simulink model "control_experiment"  (R2023b)
settings: Solver=VariableStepAuto  StartTime=0.0  StopTime=40  MaxStep=1e-4  RelTol=1e-3
values from neighbouring files (symbols this model uses):
  Bp_ = 1.25e-5    (= 1.25e-05)    [DC_motor_and_Rod.m]    (also in linearized_mechanical_model.m = 0)
  Br = 0    [DC_motor_and_Rod.m]
  c_poles = [0]    [DC_motor_and_Rod.m]
  c_zeros = [-2.121]    [DC_motor_and_Rod.m]
  g_ = 9.81    [DC_motor_and_Rod.m]    (also in linearized_mechanical_model.m)
  Jm = 4e-6 + 0.6e-6    (= 4.6e-06)    [DC_motor_and_Rod.m]
  Jp_ = (1/12)*mp_*(3*rp^2 + Lp^2)    (= 3.3718538025e-05)    [DC_motor_and_Rod.m]    (also in linearized_mechanical_model.m = 2.44e-05)
  Jr = 9.5e-5    (= 9.5e-05)    [DC_motor_and_Rod.m]
  Jr_ex_ = 9.5e-5 + Jm    (= 9.96e-05)    [DC_motor_and_Rod.m]    (also in linearized_mechanical_model.m = 9.5e-05)
  ka1 = 50    [DC_motor_and_Rod.m]
  kb1 = 5    [DC_motor_and_Rod.m]
  Kc = 0.042    [DC_motor_and_Rod.m]
  Kc_ = 0.042    [DC_motor_and_Rod.m]    (also in linearized_mechanical_model.m)
  Ke_ = 0.042    [DC_motor_and_Rod.m]    (also in linearized_mechanical_model.m)
  L = 1.16e-3    (= 0.00116)    [DC_motor_and_Rod.m]
  lp_ = 0.95*Lp/2    (= 0.061275)    [DC_motor_and_Rod.m]    (also in linearized_mechanical_model.m = 0.0645)
  Lr_ = 0.09    [DC_motor_and_Rod.m]    (also in linearized_mechanical_model.m = 0.085)
  mp_ = 0.02421    [DC_motor_and_Rod.m]    (also in linearized_mechanical_model.m = 0.024)
  Ra = 8.4    [DC_motor_and_Rod.m]
  Ra_ = 8.4    [DC_motor_and_Rod.m]    (also in linearized_mechanical_model.m)
  theta_0 = 0    [DC_motor_and_Rod.m]    (also in linearized_mechanical_model.m)
  thetadot_0 = 0    [DC_motor_and_Rod.m]    (also in linearized_mechanical_model.m)
undefined symbols (not defined in the file or in its folder): ka2, kb2, kb3
libraries: cstblocks x3, slpidlib x1
settings Model: Creator=renzo  LastModifiedBy=renzo

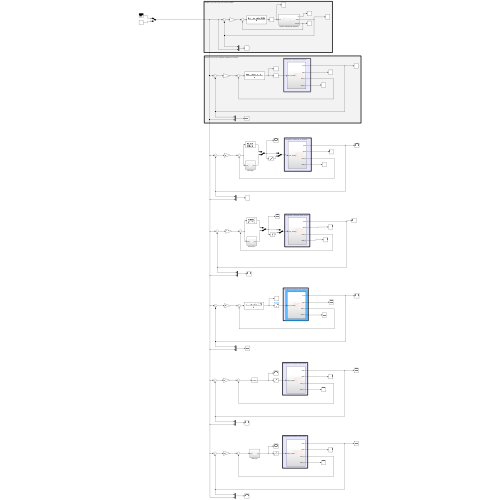
[thumbnail: Simulink's stored preview of the top-level diagram]
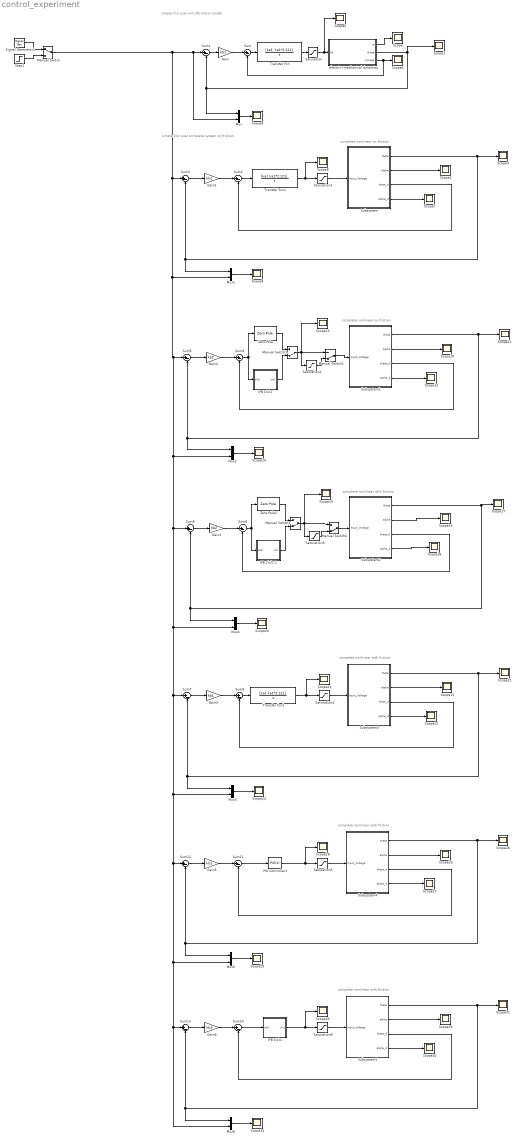
== system control_experiment ==
  note: simple C(s) over complete system no friction
  note: simple C(s) over only DC motor model
  note: complete nonlinear no friction
  note: complete nonlinear no friction
  note: complete nonlinear with friction
  note: complete nonlinear with friction
  note: complete nonlinear with friction
  note: complete nonlinear with friction
  Gain{,1,3,5} (4 alike) : Gain  Gain=kb1
  Gain2 : Gain  Gain=kb2
  Gain4 : Gain  Gain=kb2
  Gain6 : Gain  Gain=kb3
  IFB C(s)1 : Subsystem
  IFB C(s)2 : Subsystem
  IFB C(s)2.1 : Subsystem
  Manual Switch : ManualSwitch
  Manual Switch{1..4} (4 alike) : ManualSwitch  CurrentSetting=0
  Mux{,1..6} (7 alike) : Mux  Inputs=2
  PID Controller1 : slpidlib/PID Controller  Controller=PID  Form=Parallel  TimeDomain=Continuous-time  UseExternalTs=off  SampleTime=-1  IntegratorMethod=Forward Euler  FilterMethod=Forward Euler  ControllerParametersSource=internal  P=0.210656986421065  I=0.134642362226301  UseKiTs=off  D=-0.000947012474267113  N=36.4600950851827  UseFilter=on  TunerSelectOption=Transfer Function Based (PID Tuner App)  InitialConditionSource=internal  InitialConditionForIntegrator=0  InitialConditionForFilter=0  DifferentiatorICPrevScaledInput=0  ExternalReset=none  TrackingMode=off  Kt=1  LimitOutput=off  SatLimitsSource=internal  UpperSaturationLimit=inf  LowerSaturationLimit=-inf  LinearizeAsGain=on  AntiWindupMode=none  Kb=1  LimitIntegrator=off  UpperIntegratorSaturationLimit=inf  LowerIntegratorSaturationLimit=-inf  POutMin=[]  POutMax=[]  IOutMin=[]  IOutMax=[]  DOutMin=[]  DOutMax=[]  NOutMin=[]  NOutMax=[]  SumOutMin=[]  SumOutMax=[]  SaturationOutMin=[]  SaturationOutMax=[]  PParamMin=[]  PParamMax=[]  IParamMin=[]  IParamMax=[]  DParamMin=[]  DParamMax=[]  NParamMin=[]  NParamMax=[]  KbParamMin=[]  KbParamMax=[]  KtParamMin=[]  KtParamMax=[]  KbOutMin=[]  KbOutMax=[]  KtOutMin=[]  KtOutMax=[]  IntegratorOutMin=[]  IntegratorOutMax=[]  FilterOutMin=[]  FilterOutMax=[]  SumI1OutMin=[]  SumI1OutMax=[]  SumI2OutMin=[]  SumI2OutMax=[]  SumI3OutMin=[]  SumI3OutMax=[]  SumI4OutMin=[]  SumI4OutMax=[]  SumDOutMin=[]  SumDOutMax=[]  DifferentiatorOutMin=[]  DifferentiatorOutMax=[]  FilterDiffOutCoefMin=[]  FilterDiffOutCoefMax=[]  ReciprocalOutMin=[]  ReciprocalOutMax=[]  SumDenOutMin=[]  SumDenOutMax=[]  SumNumOutMin=[]  SumNumOutMax=[]  DivideOutMin=[]  DivideOutMax=[]  UdiffTsProdOutMin=[]  UdiffTsProdOutMax=[]  NTsProdOutMin=[]  NTsProdOutMax=[]  UintegralTsProdOutMin=[]  UintegralTsProdOutMax=[]  UngainTsProdOutMin=[]  UngainTsProdOutMax=[]  ClampingZeroOutDataTypeStr=Inherit: Inherit via back propagation  ClampingZeroOutMin=[]  ClampingZeroOutMax=[]  FilterDenConstantOutDataTypeStr=Inherit: Inherit via back propagation  FilterDenConstantOutMin=[]  FilterDenConstantOutMax=[]  PCopyOutDataTypeStr=Inherit: Inherit via back propagation  PCopyOutMin=[]  PCopyOutMax=[]  NCopyOutDataTypeStr=Inherit: Inherit via back propagation  NCopyOutMin=[]  NCopyOutMax=[]  IntegratorContinuousStateAttributes=''  IntegratorStateMustResolveToSignalObject=off  IntegratorRTWStateStorageClass=Auto  FilterContinuousStateAttributes=''  FilterStateMustResolveToSignalObject=off  FilterRTWStateStorageClass=Auto  ParallelPVariant=InternalParameters  IdealPVariant=Disabled  IVariant=InternalParameters  DVariant=InternalParameters  IntegratorVariant=Continuous  SatVariant=Disabled  AWVariant=Passthrough  PCopyVariant=Disabled  TRVariant=Disabled  FdbkBlocksVariant=Forward  IdealPFdbkVariant=Disabled  SatFdbkVariant=Disabled  DerivativeFilterVariant=ContFilter  NVariant=InternalParameters  NCopyVariant=Disabled  FilterICVariant=InternalICsFilter  IntegratorICVariant=InternalICs  ExternalResetVariant=Disabled  TRSumVariant=Passthrough  SumFdbkVariant=Disabled  SumVariant=Sum_PID  TsampFilterVariant=InternalTs  TsampNgainVariant=Passthrough  TsampIntegralVariant=Disabled_SignalSpec  ExternalSaturationOutDataTypeStr=Inherit: Same as second input
  Saturation{,1..6} (7 alike) : Saturate  UpperLimit=10  LowerLimit=-10
  Scope{,1..34} (35 alike) : Scope
  Signal Generator1 : SignalGenerator  WaveForm=square  Amplitude=pi/2  Frequency=0.5  Units=rad/sec
  Step1 : Step  Time=0  Before=theta_0  After=pi/2  SampleTime=0
  Subsystem : Subsystem
  Subsystem1 : Subsystem
  Subsystem2 : Subsystem
  Subsystem3 : Subsystem
  Subsystem4 : Subsystem
  Subsystem5 : Subsystem
  Sum{,1..13} (14 alike) : Sum  Inputs=|+-
  Transfer Fcn : TransferFcn  Numerator="[ka1  ka1*2.121]"  Denominator="[1  0]"
  Transfer Fcn1 : TransferFcn  Numerator=[ka1 ka1*2.121]  Denominator=[1 0]
  Transfer Fcn2 : TransferFcn  Numerator=[ka1 ka1*2.121]  Denominator=[1 0]
  Zero-Pole : ZeroPole  Zeros=c_zeros  Poles=c_poles  Gain=ka2
  Zero-Pole2 : ZeroPole  Zeros=c_zeros  Poles=c_poles  Gain=ka2
  electric+mechanical dynamics : Subsystem
  wires:
  electric+mechanical dynamics/1(ia) -> Scope/1
  Transfer Fcn/1 -> Saturation/1
  Sum/1 -> Transfer Fcn/1
  Gain/1 -> Sum/1
  Sum1/1 -> Gain/1
  electric+mechanical dynamics/2(theta) -> Scope1/1, Mux/1, Sum1/2
  Mux/1 -> Scope6/1
  electric+mechanical dynamics/3(omega) -> Sum/2, Scope4/1
  Step1/1 -> Manual Switch/2
  Signal Generator1/1 -> Manual Switch/1
  Mux1/1 -> Scope9/1
  Sum2/1 -> Transfer Fcn1/1
  Sum3/1 -> Gain1/1
  Subsystem/1(theta) -> Scope3/1, Sum3/2, Mux1/1
  Gain1/1 -> Sum2/1
  Subsystem/2(alpha) -> Scope2/1
  Subsystem/3(theta_d) -> Sum2/2
  Subsystem/4(alpha_d) -> Scope7/1
  Saturation/1 -> Scope5/1, electric+mechanical dynamics/1(Va)
  Saturation1/1 -> Subsystem/1(Input_Voltage)
  Transfer Fcn1/1 -> Scope8/1, Saturation1/1
  Manual Switch1/1 -> Saturation2/1, Manual Switch2/1, Scope13/1
  Subsystem1/1(theta) -> Scope11/1, Sum5/2, Mux2/1
  Subsystem1/2(alpha) -> Scope10/1
  Gain2/1 -> Sum4/1
  Subsystem1/3(theta_d) -> Sum4/2
  Sum4/1 -> IFB C(s)2/1(e(s)), Zero-Pole/1
  Sum5/1 -> Gain2/1
  Mux2/1 -> Scope14/1
  Subsystem1/4(alpha_d) -> Scope12/1
  IFB C(s)2/1(u(s)) -> Manual Switch1/2
  Zero-Pole/1 -> Manual Switch1/1
  Saturation2/1 -> Manual Switch2/2
  Manual Switch2/1 -> Subsystem1/1(Input_Voltage)
  Subsystem2/2(alpha) -> Scope16/1
  Subsystem2/4(alpha_d) -> Scope18/1
  Subsystem2/3(theta_d) -> Sum8/2
  Gain4/1 -> Sum8/1
  Saturation3/1 -> Manual Switch4/2
  IFB C(s)2.1/1(u(s)) -> Manual Switch3/2
  Zero-Pole2/1 -> Manual Switch3/1
  Sum9/1 -> Gain4/1
  Sum8/1 -> IFB C(s)2.1/1(e(s)), Zero-Pole2/1
  Mux4/1 -> Scope20/1
  Manual Switch3/1 -> Saturation3/1, Manual Switch4/1, Scope19/1
  Subsystem2/1(theta) -> Sum9/2, Mux4/1, Scope17/1
  Manual Switch4/1 -> Subsystem2/1(Input_Voltage)
  Saturation4/1 -> Subsystem3/1(Input_Voltage)
  Subsystem3/4(alpha_d) -> Scope22/1
  Sum6/1 -> Transfer Fcn2/1
  Gain3/1 -> Sum6/1
  Mux3/1 -> Scope24/1
  Transfer Fcn2/1 -> Scope23/1, Saturation4/1
  Subsystem3/2(alpha) -> Scope15/1
  Sum7/1 -> Gain3/1
  Subsystem3/3(theta_d) -> Sum6/2
  Subsystem3/1(theta) -> Scope21/1, Sum7/2, Mux3/1
  Subsystem4/1(theta) -> Scope26/1, Sum12/2, Mux5/1
  Subsystem4/3(theta_d) -> Sum11/2
  Sum12/1 -> Gain5/1
  Gain5/1 -> Sum11/1
  Mux5/1 -> Scope29/1
  Sum11/1 -> PID Controller1/1
  PID Controller1/1 -> Scope28/1, Saturation5/1
  Subsystem4/2(alpha) -> Scope25/1
  Saturation5/1 -> Subsystem4/1(Input_Voltage)
  Subsystem4/4(alpha_d) -> Scope27/1
  Subsystem5/4(alpha_d) -> Scope32/1
  Saturation6/1 -> Subsystem5/1(Input_Voltage)
  Sum10/1 -> IFB C(s)1/1(e(s))
  IFB C(s)1/1(u(s)) -> Scope33/1, Saturation6/1
  Sum13/1 -> Gain6/1
  Subsystem5/2(alpha) -> Scope30/1
  Manual Switch/1 -> Mux1/2, Mux3/2, Mux6/2, Sum13/1, Mux5/2, Sum12/1, Sum7/1, Mux4/2, Sum9/1, Mux2/2, Sum5/1, Sum3/1, Sum1/1, Mux/2
  Mux6/1 -> Scope34/1
  Subsystem5/3(theta_d) -> Sum10/2
  Gain6/1 -> Sum10/1
  Subsystem5/1(theta) -> Scope31/1, Sum13/2, Mux6/1

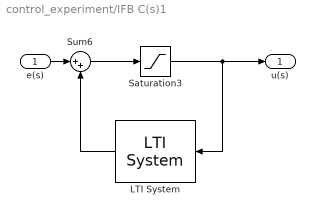
== system control_experiment/IFB C(s)1 ==
  e(s) : Inport
  LTI System : cstblocks/LTI System  sys=Hs3  IC=[]  PadeOrder=0
  Saturation3 : Saturate  UpperLimit=10  LowerLimit=-10
  Sum6 : Sum  Inputs=|++
  u(s) : Outport
  wires:
  e(s)/1 -> Sum6/1
  Saturation3/1 -> LTI System/1, u(s)/1
  Sum6/1 -> Saturation3/1
  LTI System/1 -> Sum6/2

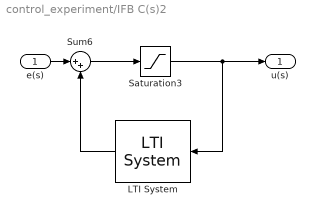
== system control_experiment/IFB C(s)2 ==
  e(s) : Inport
  LTI System : cstblocks/LTI System  sys=Hs2  IC=[]  PadeOrder=0
  Saturation3 : Saturate  UpperLimit=10  LowerLimit=-10
  Sum6 : Sum  Inputs=|++
  u(s) : Outport
  wires:
  LTI System/1 -> Sum6/2
  Sum6/1 -> Saturation3/1
  Saturation3/1 -> u(s)/1, LTI System/1
  e(s)/1 -> Sum6/1

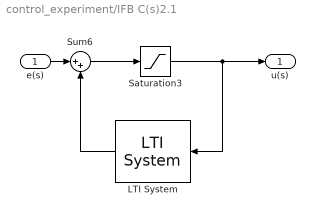
== system control_experiment/IFB C(s)2.1 ==
  e(s) : Inport
  LTI System : cstblocks/LTI System  sys=Hs2  IC=[]  PadeOrder=0
  Saturation3 : Saturate  UpperLimit=10  LowerLimit=-10
  Sum6 : Sum  Inputs=|++
  u(s) : Outport
  wires:
  LTI System/1 -> Sum6/2
  Sum6/1 -> Saturation3/1
  Saturation3/1 -> u(s)/1, LTI System/1
  e(s)/1 -> Sum6/1

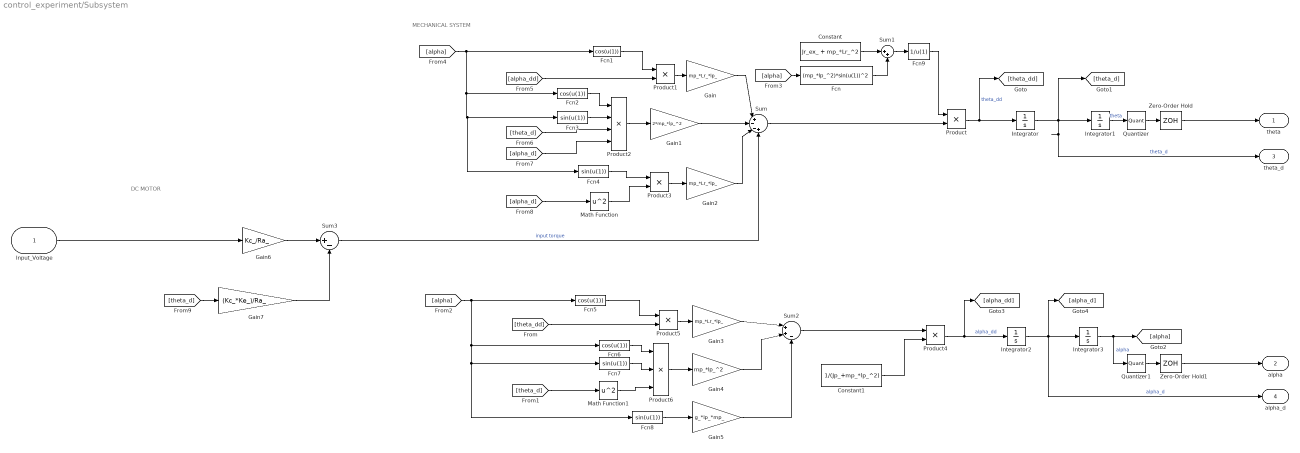
== system control_experiment/Subsystem ==
  note: DC MOTOR
  note: MECHANICAL SYSTEM
  Input_Voltage : Inport
  Constant : Constant  Value=Jr_ex_ + mp_*Lr_^2
  Constant1 : Constant  Value=1/(Jp_+mp_*lp_^2)
  Fcn : Fcn  Expr=(mp_*lp_^2)*sin(u(1))^2
  Fcn{1..2,5..6} (4 alike) : Fcn  Expr=cos(u(1))
  Fcn{3..4,7..8} (4 alike) : Fcn  Expr=sin(u(1))
  Fcn9 : Fcn  Expr=1/u(1)
  Gain : Gain  Gain=mp_*Lr_*lp_
  Gain1 : Gain  Gain=2*mp_*lp_^2
  Gain2 : Gain  Gain=mp_*Lr_*lp_
  Gain3 : Gain  Gain=mp_*Lr_*lp_
  Gain4 : Gain  Gain=mp_*lp_^2
  Gain5 : Gain  Gain=g_*lp_*mp_
  Gain6 : Gain  Gain=Kc_/Ra_
  Gain7 : Gain  Gain=(Kc_*Ke_)/Ra_
  Integrator : Integrator
  Integrator1 : Integrator  InitialCondition=theta_0
  Integrator2 : Integrator
  Integrator3 : Integrator
  Math Function : Math  Operator=square
  Math Function1 : Math  Operator=square
  Product{,1,3..5} (5 alike) : Product
  Product2 : Product  Inputs=4
  Product6 : Product  Inputs=3
  Quantizer : Quantizer  QuantizationInterval=0.0037
  Quantizer1 : Quantizer  QuantizationInterval=0.0037
  Sum : Sum  Inputs=|+--+
  Sum1 : Sum  Inputs=|++
  Sum2 : Sum  Inputs=|++-
  Sum3 : Sum  Inputs=|+-
  Zero-Order Hold : ZeroOrderHold  SampleTime=2e-3
  Zero-Order Hold1 : ZeroOrderHold  SampleTime=2e-3
  theta : Outport
  alpha : Outport  Port=2
  theta_d : Outport  Port=3
  alpha_d : Outport  Port=4
  wires:
  Integrator2/1 -> alpha_d/1, Integrator3/1, [alpha_d]  "alpha_d"
  Fcn6/1 -> Product6/1
  Product4/1 -> [alpha_dd], Integrator2/1  "alpha_dd"
  Fcn4/1 -> Product3/1
  Integrator/1 -> theta_d/1, [theta_d], Integrator1/1  "theta_d"
  Gain1/1 -> Sum/2
  Gain6/1 -> Sum3/1
  Fcn3/1 -> Product2/2
  Fcn1/1 -> Product1/1
  Fcn8/1 -> Gain5/1
  Fcn7/1 -> Product6/2
  Gain5/1 -> Sum2/3
  Sum1/1 -> Fcn9/1
  Fcn/1 -> Sum1/2
  Product1/1 -> Gain/1
  Fcn9/1 -> Product/1
  Product3/1 -> Gain2/1
  Sum/1 -> Product/2
  [alpha_d] -> Math Function/1
  [theta_dd] -> Product5/2
  [theta_d] -> Gain7/1
  Product5/1 -> Gain3/1
  Integrator3/1 -> Quantizer1/1, [alpha]  "alpha"
  Fcn5/1 -> Product5/1
  Product6/1 -> Gain4/1
  Sum2/1 -> Product4/1
  Math Function1/1 -> Product6/3
  Math Function/1 -> Product3/2
  Product/1 -> Integrator/1, [theta_dd]  "theta_dd"
  Gain4/1 -> Sum2/2
  Input_Voltage/1 -> Gain6/1
  Constant/1 -> Sum1/1
  [alpha] -> Fcn8/1, Fcn7/1, Fcn6/1, Fcn5/1
  Constant1/1 -> Product4/2
  Product2/1 -> Gain1/1
  [alpha] -> Fcn4/1, Fcn3/1, Fcn2/1, Fcn1/1
  [alpha_d] -> Product2/4
  [alpha_dd] -> Product1/2
  [alpha] -> Fcn/1
  Fcn2/1 -> Product2/1
  Sum3/1 -> Sum/4  "input torque"
  Gain2/1 -> Sum/3
  Gain/1 -> Sum/1
  Gain3/1 -> Sum2/1
  [theta_d] -> Math Function1/1
  Gain7/1 -> Sum3/2
  [theta_d] -> Product2/3
  Integrator1/1 -> Quantizer/1  "theta"
  Quantizer/1 -> Zero-Order Hold/1
  Zero-Order Hold/1 -> theta/1
  Quantizer1/1 -> Zero-Order Hold1/1
  Zero-Order Hold1/1 -> alpha/1

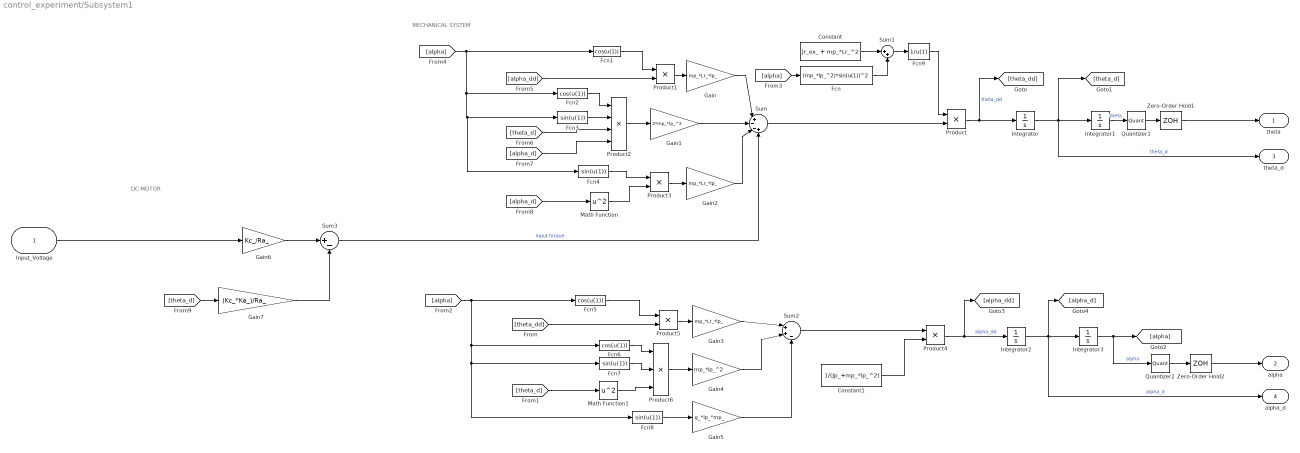
== system control_experiment/Subsystem1 ==
  note: DC MOTOR
  note: MECHANICAL SYSTEM
  Input_Voltage : Inport
  Constant : Constant  Value=Jr_ex_ + mp_*Lr_^2
  Constant1 : Constant  Value=1/(Jp_+mp_*lp_^2)
  Fcn : Fcn  Expr=(mp_*lp_^2)*sin(u(1))^2
  Fcn{1..2,5..6} (4 alike) : Fcn  Expr=cos(u(1))
  Fcn{3..4,7..8} (4 alike) : Fcn  Expr=sin(u(1))
  Fcn9 : Fcn  Expr=1/u(1)
  Gain : Gain  Gain=mp_*Lr_*lp_
  Gain1 : Gain  Gain=2*mp_*lp_^2
  Gain2 : Gain  Gain=mp_*Lr_*lp_
  Gain3 : Gain  Gain=mp_*Lr_*lp_
  Gain4 : Gain  Gain=mp_*lp_^2
  Gain5 : Gain  Gain=g_*lp_*mp_
  Gain6 : Gain  Gain=Kc_/Ra_
  Gain7 : Gain  Gain=(Kc_*Ke_)/Ra_
  Integrator : Integrator
  Integrator1 : Integrator  InitialCondition=theta_0
  Integrator2 : Integrator
  Integrator3 : Integrator
  Math Function : Math  Operator=square
  Math Function1 : Math  Operator=square
  Product{,1,3..5} (5 alike) : Product
  Product2 : Product  Inputs=4
  Product6 : Product  Inputs=3
  Quantizer1 : Quantizer  QuantizationInterval=0.0037
  Quantizer2 : Quantizer  QuantizationInterval=0.0037
  Sum : Sum  Inputs=|+--+
  Sum1 : Sum  Inputs=|++
  Sum2 : Sum  Inputs=|++-
  Sum3 : Sum  Inputs=|+-
  Zero-Order Hold1 : ZeroOrderHold  SampleTime=2e-3
  Zero-Order Hold2 : ZeroOrderHold  SampleTime=2e-3
  theta : Outport
  alpha : Outport  Port=2
  theta_d : Outport  Port=3
  alpha_d : Outport  Port=4
  wires:
  Integrator2/1 -> alpha_d/1, Integrator3/1, [alpha_d]  "alpha_d"
  Fcn6/1 -> Product6/1
  Product4/1 -> [alpha_dd], Integrator2/1  "alpha_dd"
  Fcn4/1 -> Product3/1
  Integrator/1 -> theta_d/1, [theta_d], Integrator1/1  "theta_d"
  Gain1/1 -> Sum/2
  Gain6/1 -> Sum3/1
  Fcn3/1 -> Product2/2
  Fcn1/1 -> Product1/1
  Integrator1/1 -> Quantizer1/1  "theta"
  Fcn8/1 -> Gain5/1
  Fcn7/1 -> Product6/2
  Gain5/1 -> Sum2/3
  Sum1/1 -> Fcn9/1
  Fcn/1 -> Sum1/2
  Product1/1 -> Gain/1
  Fcn9/1 -> Product/1
  Product3/1 -> Gain2/1
  Sum/1 -> Product/2
  [alpha_d] -> Math Function/1
  [theta_dd] -> Product5/2
  [theta_d] -> Gain7/1
  Product5/1 -> Gain3/1
  Integrator3/1 -> Quantizer2/1, [alpha]  "alpha"
  Fcn5/1 -> Product5/1
  Product6/1 -> Gain4/1
  Sum2/1 -> Product4/1
  Math Function1/1 -> Product6/3
  Math Function/1 -> Product3/2
  Product/1 -> Integrator/1, [theta_dd]  "theta_dd"
  Gain4/1 -> Sum2/2
  Input_Voltage/1 -> Gain6/1
  Constant/1 -> Sum1/1
  [alpha] -> Fcn8/1, Fcn7/1, Fcn6/1, Fcn5/1
  Constant1/1 -> Product4/2
  Product2/1 -> Gain1/1
  [alpha] -> Fcn4/1, Fcn3/1, Fcn2/1, Fcn1/1
  [alpha_d] -> Product2/4
  [alpha_dd] -> Product1/2
  [alpha] -> Fcn/1
  Fcn2/1 -> Product2/1
  Sum3/1 -> Sum/4  "input torque"
  Gain2/1 -> Sum/3
  Gain/1 -> Sum/1
  Gain3/1 -> Sum2/1
  [theta_d] -> Math Function1/1
  Gain7/1 -> Sum3/2
  [theta_d] -> Product2/3
  Quantizer1/1 -> Zero-Order Hold1/1
  Zero-Order Hold1/1 -> theta/1
  Quantizer2/1 -> Zero-Order Hold2/1
  Zero-Order Hold2/1 -> alpha/1

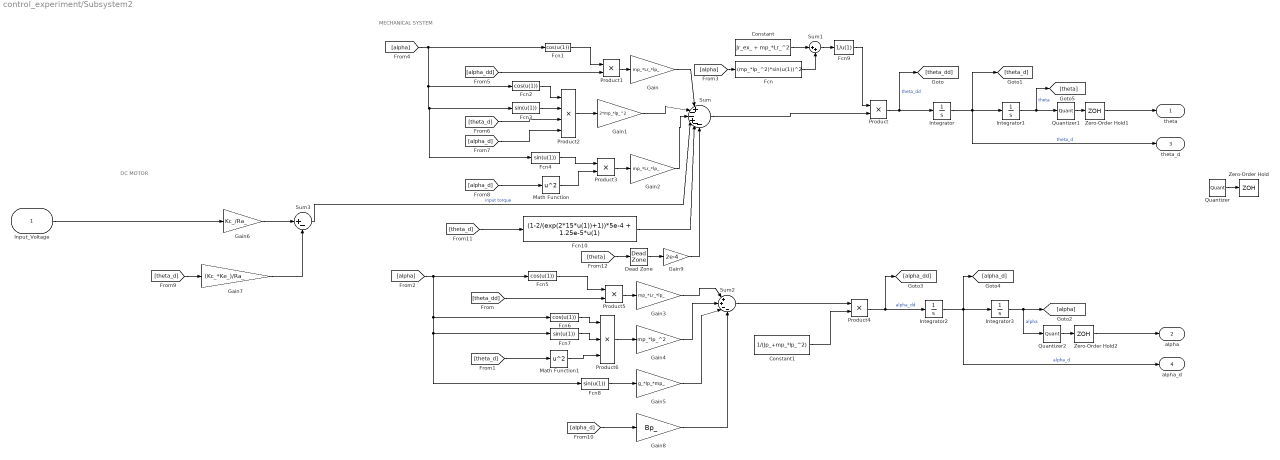
== system control_experiment/Subsystem2 ==
  note: MECHANICAL SYSTEM
  note: DC MOTOR
  Input_Voltage : Inport
  Constant : Constant  Value=Jr_ex_ + mp_*Lr_^2
  Constant1 : Constant  Value=1/(Jp_+mp_*lp_^2)
  Dead Zone : DeadZone  LowerValue=0  UpperValue=0  ZeroCross=off
  Fcn : Fcn  Expr=(mp_*lp_^2)*sin(u(1))^2
  Fcn{1..2,5..6} (4 alike) : Fcn  Expr=cos(u(1))
  Fcn10 : Fcn  Expr=(1-2/(exp(2*15*u(1))+1))*5e-4 + 1.25e-5*u(1)
  Fcn{3..4,7..8} (4 alike) : Fcn  Expr=sin(u(1))
  Fcn9 : Fcn  Expr=1/u(1)
  Gain : Gain  Gain=mp_*Lr_*lp_
  Gain1 : Gain  Gain=2*mp_*lp_^2
  Gain2 : Gain  Gain=mp_*Lr_*lp_
  Gain3 : Gain  Gain=mp_*Lr_*lp_
  Gain4 : Gain  Gain=mp_*lp_^2
  Gain5 : Gain  Gain=g_*lp_*mp_
  Gain6 : Gain  Gain=Kc_/Ra_
  Gain7 : Gain  Gain=(Kc_*Ke_)/Ra_
  Gain8 : Gain  Gain=Bp_
  Gain9 : Gain  Gain=2e-4
  Integrator{,1..3} (4 alike) : Integrator
  Math Function : Math  Operator=square
  Math Function1 : Math  Operator=square
  Product{,1,3..5} (5 alike) : Product
  Product2 : Product  Inputs=4
  Product6 : Product  Inputs=3
  Quantizer : Quantizer  QuantizationInterval=0.0037
  Quantizer1 : Quantizer  QuantizationInterval=0.0037
  Quantizer2 : Quantizer  QuantizationInterval=0.0037
  Sum : Sum  Inputs=|+--+--
  Sum1 : Sum  Inputs=|++
  Sum2 : Sum  Inputs=|++--
  Sum3 : Sum  Inputs=|+-
  Zero-Order Hold : ZeroOrderHold  SampleTime=2e-3
  Zero-Order Hold1 : ZeroOrderHold  SampleTime=2e-3
  Zero-Order Hold2 : ZeroOrderHold  SampleTime=2e-3
  theta : Outport
  alpha : Outport  Port=2
  theta_d : Outport  Port=3
  alpha_d : Outport  Port=4
  wires:
  [theta_d] -> Product2/3
  Gain7/1 -> Sum3/2
  [theta_d] -> Math Function1/1
  Gain3/1 -> Sum2/1
  Gain/1 -> Sum/1
  Gain2/1 -> Sum/3
  Sum3/1 -> Sum/4  "input torque"
  Fcn2/1 -> Product2/1
  [alpha] -> Fcn/1
  [alpha_dd] -> Product1/2
  [alpha_d] -> Product2/4
  [alpha] -> Fcn1/1, Fcn2/1, Fcn3/1, Fcn4/1
  Product2/1 -> Gain1/1
  Constant1/1 -> Product4/2
  [alpha] -> Fcn5/1, Fcn6/1, Fcn7/1, Fcn8/1
  Constant/1 -> Sum1/1
  Input_Voltage/1 -> Gain6/1
  Gain4/1 -> Sum2/2
  Product/1 -> [theta_dd], Integrator/1  "theta_dd"
  Math Function/1 -> Product3/2
  Math Function1/1 -> Product6/3
  Sum2/1 -> Product4/1
  Product6/1 -> Gain4/1
  Fcn5/1 -> Product5/1
  Integrator3/1 -> [alpha], Quantizer2/1  "alpha"
  Product5/1 -> Gain3/1
  [theta_d] -> Gain7/1
  [theta_dd] -> Product5/2
  [alpha_d] -> Math Function/1
  Sum/1 -> Product/2
  Product3/1 -> Gain2/1
  Fcn9/1 -> Product/1
  Product1/1 -> Gain/1
  Fcn/1 -> Sum1/2
  Sum1/1 -> Fcn9/1
  Gain5/1 -> Sum2/3
  Fcn7/1 -> Product6/2
  Fcn8/1 -> Gain5/1
  Integrator1/1 -> Quantizer1/1, [theta]  "theta"
  Fcn1/1 -> Product1/1
  Fcn3/1 -> Product2/2
  Gain6/1 -> Sum3/1
  Gain1/1 -> Sum/2
  Integrator/1 -> Integrator1/1, [theta_d], theta_d/1  "theta_d"
  Fcn4/1 -> Product3/1
  Product4/1 -> Integrator2/1, [alpha_dd]  "alpha_dd"
  Fcn6/1 -> Product6/1
  Integrator2/1 -> [alpha_d], Integrator3/1, alpha_d/1  "alpha_d"
  [alpha_d] -> Gain8/1
  Gain8/1 -> Sum2/4
  [theta_d] -> Fcn10/1
  Dead Zone/1 -> Gain9/1
  Gain9/1 -> Sum/6
  [theta] -> Dead Zone/1
  Fcn10/1 -> Sum/5
  Quantizer/1 -> Zero-Order Hold/1
  ? -> Quantizer/1  "theta"
  Quantizer1/1 -> Zero-Order Hold1/1
  Zero-Order Hold1/1 -> theta/1
  Quantizer2/1 -> Zero-Order Hold2/1
  Zero-Order Hold2/1 -> alpha/1

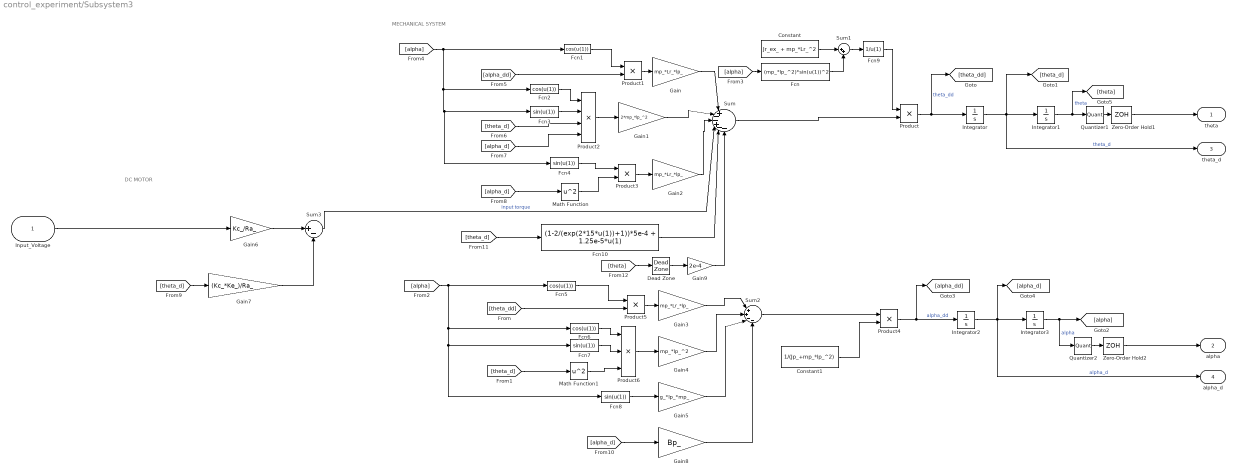
== system control_experiment/Subsystem3 ==
  note: DC MOTOR
  note: MECHANICAL SYSTEM
  Input_Voltage : Inport
  Constant : Constant  Value=Jr_ex_ + mp_*Lr_^2
  Constant1 : Constant  Value=1/(Jp_+mp_*lp_^2)
  Dead Zone : DeadZone  LowerValue=0  UpperValue=0  ZeroCross=off
  Fcn : Fcn  Expr=(mp_*lp_^2)*sin(u(1))^2
  Fcn{1..2,5..6} (4 alike) : Fcn  Expr=cos(u(1))
  Fcn10 : Fcn  Expr=(1-2/(exp(2*15*u(1))+1))*5e-4 + 1.25e-5*u(1)
  Fcn{3..4,7..8} (4 alike) : Fcn  Expr=sin(u(1))
  Fcn9 : Fcn  Expr=1/u(1)
  Gain : Gain  Gain=mp_*Lr_*lp_
  Gain1 : Gain  Gain=2*mp_*lp_^2
  Gain2 : Gain  Gain=mp_*Lr_*lp_
  Gain3 : Gain  Gain=mp_*Lr_*lp_
  Gain4 : Gain  Gain=mp_*lp_^2
  Gain5 : Gain  Gain=g_*lp_*mp_
  Gain6 : Gain  Gain=Kc_/Ra_
  Gain7 : Gain  Gain=(Kc_*Ke_)/Ra_
  Gain8 : Gain  Gain=Bp_
  Gain9 : Gain  Gain=2e-4
  Integrator{,1..3} (4 alike) : Integrator
  Math Function : Math  Operator=square
  Math Function1 : Math  Operator=square
  Product{,1,3..5} (5 alike) : Product
  Product2 : Product  Inputs=4
  Product6 : Product  Inputs=3
  Quantizer1 : Quantizer  QuantizationInterval=0.0037
  Quantizer2 : Quantizer  QuantizationInterval=0.0037
  Sum : Sum  Inputs=|+--+--
  Sum1 : Sum  Inputs=|++
  Sum2 : Sum  Inputs=|++--
  Sum3 : Sum  Inputs=|+-
  Zero-Order Hold1 : ZeroOrderHold  SampleTime=2e-3
  Zero-Order Hold2 : ZeroOrderHold  SampleTime=2e-3
  theta : Outport
  alpha : Outport  Port=2
  theta_d : Outport  Port=3
  alpha_d : Outport  Port=4
  wires:
  Fcn10/1 -> Sum/5
  [theta] -> Dead Zone/1
  Gain9/1 -> Sum/6
  Dead Zone/1 -> Gain9/1
  [theta_d] -> Fcn10/1
  Gain8/1 -> Sum2/4
  [alpha_d] -> Gain8/1
  Integrator2/1 -> alpha_d/1, Integrator3/1, [alpha_d]  "alpha_d"
  Fcn6/1 -> Product6/1
  Product4/1 -> [alpha_dd], Integrator2/1  "alpha_dd"
  Fcn4/1 -> Product3/1
  Integrator/1 -> theta_d/1, [theta_d], Integrator1/1  "theta_d"
  Gain1/1 -> Sum/2
  Gain6/1 -> Sum3/1
  Fcn3/1 -> Product2/2
  Fcn1/1 -> Product1/1
  Integrator1/1 -> [theta], Quantizer1/1  "theta"
  Fcn8/1 -> Gain5/1
  Fcn7/1 -> Product6/2
  Gain5/1 -> Sum2/3
  Sum1/1 -> Fcn9/1
  Fcn/1 -> Sum1/2
  Product1/1 -> Gain/1
  Fcn9/1 -> Product/1
  Product3/1 -> Gain2/1
  Sum/1 -> Product/2
  [alpha_d] -> Math Function/1
  [theta_dd] -> Product5/2
  [theta_d] -> Gain7/1
  Product5/1 -> Gain3/1
  Integrator3/1 -> Quantizer2/1, [alpha]  "alpha"
  Fcn5/1 -> Product5/1
  Product6/1 -> Gain4/1
  Sum2/1 -> Product4/1
  Math Function1/1 -> Product6/3
  Math Function/1 -> Product3/2
  Product/1 -> Integrator/1, [theta_dd]  "theta_dd"
  Gain4/1 -> Sum2/2
  Input_Voltage/1 -> Gain6/1
  Constant/1 -> Sum1/1
  [alpha] -> Fcn8/1, Fcn7/1, Fcn6/1, Fcn5/1
  Constant1/1 -> Product4/2
  Product2/1 -> Gain1/1
  [alpha] -> Fcn4/1, Fcn3/1, Fcn2/1, Fcn1/1
  [alpha_d] -> Product2/4
  [alpha_dd] -> Product1/2
  [alpha] -> Fcn/1
  Fcn2/1 -> Product2/1
  Sum3/1 -> Sum/4  "input torque"
  Gain2/1 -> Sum/3
  Gain/1 -> Sum/1
  Gain3/1 -> Sum2/1
  [theta_d] -> Math Function1/1
  Gain7/1 -> Sum3/2
  [theta_d] -> Product2/3
  Zero-Order Hold1/1 -> theta/1
  Quantizer2/1 -> Zero-Order Hold2/1
  Zero-Order Hold2/1 -> alpha/1
  Quantizer1/1 -> Zero-Order Hold1/1

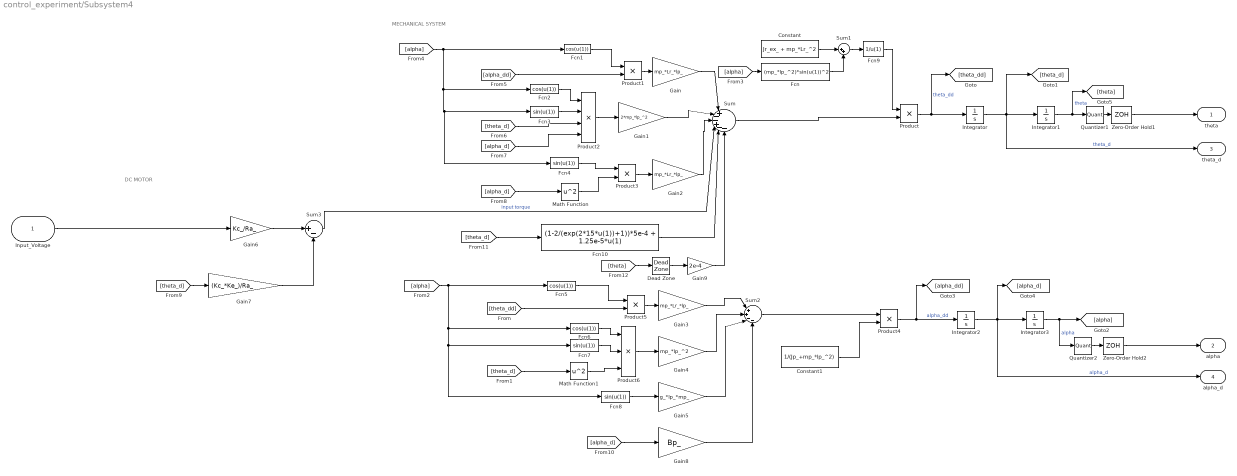
== system control_experiment/Subsystem4 ==
  note: DC MOTOR
  note: MECHANICAL SYSTEM
  Input_Voltage : Inport
  Constant : Constant  Value=Jr_ex_ + mp_*Lr_^2
  Constant1 : Constant  Value=1/(Jp_+mp_*lp_^2)
  Dead Zone : DeadZone  LowerValue=0  UpperValue=0  ZeroCross=off
  Fcn : Fcn  Expr=(mp_*lp_^2)*sin(u(1))^2
  Fcn{1..2,5..6} (4 alike) : Fcn  Expr=cos(u(1))
  Fcn10 : Fcn  Expr=(1-2/(exp(2*15*u(1))+1))*5e-4 + 1.25e-5*u(1)
  Fcn{3..4,7..8} (4 alike) : Fcn  Expr=sin(u(1))
  Fcn9 : Fcn  Expr=1/u(1)
  Gain : Gain  Gain=mp_*Lr_*lp_
  Gain1 : Gain  Gain=2*mp_*lp_^2
  Gain2 : Gain  Gain=mp_*Lr_*lp_
  Gain3 : Gain  Gain=mp_*Lr_*lp_
  Gain4 : Gain  Gain=mp_*lp_^2
  Gain5 : Gain  Gain=g_*lp_*mp_
  Gain6 : Gain  Gain=Kc_/Ra_
  Gain7 : Gain  Gain=(Kc_*Ke_)/Ra_
  Gain8 : Gain  Gain=Bp_
  Gain9 : Gain  Gain=2e-4
  Integrator{,1..3} (4 alike) : Integrator
  Math Function : Math  Operator=square
  Math Function1 : Math  Operator=square
  Product{,1,3..5} (5 alike) : Product
  Product2 : Product  Inputs=4
  Product6 : Product  Inputs=3
  Quantizer1 : Quantizer  QuantizationInterval=0.0037
  Quantizer2 : Quantizer  QuantizationInterval=0.0037
  Sum : Sum  Inputs=|+--+--
  Sum1 : Sum  Inputs=|++
  Sum2 : Sum  Inputs=|++--
  Sum3 : Sum  Inputs=|+-
  Zero-Order Hold1 : ZeroOrderHold  SampleTime=2e-3
  Zero-Order Hold2 : ZeroOrderHold  SampleTime=2e-3
  theta : Outport
  alpha : Outport  Port=2
  theta_d : Outport  Port=3
  alpha_d : Outport  Port=4
  wires:
  Fcn10/1 -> Sum/5
  [theta] -> Dead Zone/1
  Gain9/1 -> Sum/6
  Dead Zone/1 -> Gain9/1
  [theta_d] -> Fcn10/1
  Gain8/1 -> Sum2/4
  [alpha_d] -> Gain8/1
  Integrator2/1 -> alpha_d/1, Integrator3/1, [alpha_d]  "alpha_d"
  Fcn6/1 -> Product6/1
  Product4/1 -> [alpha_dd], Integrator2/1  "alpha_dd"
  Fcn4/1 -> Product3/1
  Integrator/1 -> theta_d/1, [theta_d], Integrator1/1  "theta_d"
  Gain1/1 -> Sum/2
  Gain6/1 -> Sum3/1
  Fcn3/1 -> Product2/2
  Fcn1/1 -> Product1/1
  Integrator1/1 -> [theta], Quantizer1/1  "theta"
  Fcn8/1 -> Gain5/1
  Fcn7/1 -> Product6/2
  Gain5/1 -> Sum2/3
  Sum1/1 -> Fcn9/1
  Fcn/1 -> Sum1/2
  Product1/1 -> Gain/1
  Fcn9/1 -> Product/1
  Product3/1 -> Gain2/1
  Sum/1 -> Product/2
  [alpha_d] -> Math Function/1
  [theta_dd] -> Product5/2
  [theta_d] -> Gain7/1
  Product5/1 -> Gain3/1
  Integrator3/1 -> Quantizer2/1, [alpha]  "alpha"
  Fcn5/1 -> Product5/1
  Product6/1 -> Gain4/1
  Sum2/1 -> Product4/1
  Math Function1/1 -> Product6/3
  Math Function/1 -> Product3/2
  Product/1 -> Integrator/1, [theta_dd]  "theta_dd"
  Gain4/1 -> Sum2/2
  Input_Voltage/1 -> Gain6/1
  Constant/1 -> Sum1/1
  [alpha] -> Fcn8/1, Fcn7/1, Fcn6/1, Fcn5/1
  Constant1/1 -> Product4/2
  Product2/1 -> Gain1/1
  [alpha] -> Fcn4/1, Fcn3/1, Fcn2/1, Fcn1/1
  [alpha_d] -> Product2/4
  [alpha_dd] -> Product1/2
  [alpha] -> Fcn/1
  Fcn2/1 -> Product2/1
  Sum3/1 -> Sum/4  "input torque"
  Gain2/1 -> Sum/3
  Gain/1 -> Sum/1
  Gain3/1 -> Sum2/1
  [theta_d] -> Math Function1/1
  Gain7/1 -> Sum3/2
  [theta_d] -> Product2/3
  Zero-Order Hold1/1 -> theta/1
  Quantizer2/1 -> Zero-Order Hold2/1
  Zero-Order Hold2/1 -> alpha/1
  Quantizer1/1 -> Zero-Order Hold1/1

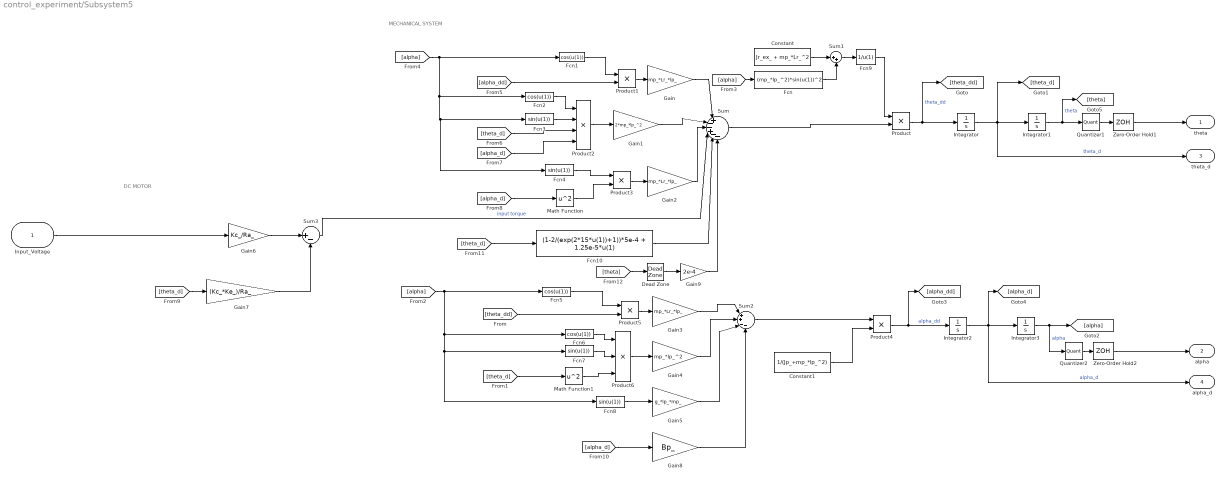
== system control_experiment/Subsystem5 ==
  note: DC MOTOR
  note: MECHANICAL SYSTEM
  Input_Voltage : Inport
  Constant : Constant  Value=Jr_ex_ + mp_*Lr_^2
  Constant1 : Constant  Value=1/(Jp_+mp_*lp_^2)
  Dead Zone : DeadZone  LowerValue=0  UpperValue=0  ZeroCross=off
  Fcn : Fcn  Expr=(mp_*lp_^2)*sin(u(1))^2
  Fcn{1..2,5..6} (4 alike) : Fcn  Expr=cos(u(1))
  Fcn10 : Fcn  Expr=(1-2/(exp(2*15*u(1))+1))*5e-4 + 1.25e-5*u(1)
  Fcn{3..4,7..8} (4 alike) : Fcn  Expr=sin(u(1))
  Fcn9 : Fcn  Expr=1/u(1)
  Gain : Gain  Gain=mp_*Lr_*lp_
  Gain1 : Gain  Gain=2*mp_*lp_^2
  Gain2 : Gain  Gain=mp_*Lr_*lp_
  Gain3 : Gain  Gain=mp_*Lr_*lp_
  Gain4 : Gain  Gain=mp_*lp_^2
  Gain5 : Gain  Gain=g_*lp_*mp_
  Gain6 : Gain  Gain=Kc_/Ra_
  Gain7 : Gain  Gain=(Kc_*Ke_)/Ra_
  Gain8 : Gain  Gain=Bp_
  Gain9 : Gain  Gain=2e-4
  Integrator{,1..3} (4 alike) : Integrator
  Math Function : Math  Operator=square
  Math Function1 : Math  Operator=square
  Product{,1,3..5} (5 alike) : Product
  Product2 : Product  Inputs=4
  Product6 : Product  Inputs=3
  Quantizer1 : Quantizer  QuantizationInterval=0.0037
  Quantizer2 : Quantizer  QuantizationInterval=0.0037
  Sum : Sum  Inputs=|+--+--
  Sum1 : Sum  Inputs=|++
  Sum2 : Sum  Inputs=|++--
  Sum3 : Sum  Inputs=|+-
  Zero-Order Hold1 : ZeroOrderHold  SampleTime=2e-3
  Zero-Order Hold2 : ZeroOrderHold  SampleTime=2e-3
  theta : Outport
  alpha : Outport  Port=2
  theta_d : Outport  Port=3
  alpha_d : Outport  Port=4
  wires:
  Fcn10/1 -> Sum/5
  [theta] -> Dead Zone/1
  Gain9/1 -> Sum/6
  Dead Zone/1 -> Gain9/1
  [theta_d] -> Fcn10/1
  Gain8/1 -> Sum2/4
  [alpha_d] -> Gain8/1
  Integrator2/1 -> alpha_d/1, Integrator3/1, [alpha_d]  "alpha_d"
  Fcn6/1 -> Product6/1
  Product4/1 -> [alpha_dd], Integrator2/1  "alpha_dd"
  Fcn4/1 -> Product3/1
  Integrator/1 -> theta_d/1, [theta_d], Integrator1/1  "theta_d"
  Gain1/1 -> Sum/2
  Gain6/1 -> Sum3/1
  Fcn3/1 -> Product2/2
  Fcn1/1 -> Product1/1
  Integrator1/1 -> [theta], Quantizer1/1  "theta"
  Fcn8/1 -> Gain5/1
  Fcn7/1 -> Product6/2
  Gain5/1 -> Sum2/3
  Sum1/1 -> Fcn9/1
  Fcn/1 -> Sum1/2
  Product1/1 -> Gain/1
  Fcn9/1 -> Product/1
  Product3/1 -> Gain2/1
  Sum/1 -> Product/2
  [alpha_d] -> Math Function/1
  [theta_dd] -> Product5/2
  [theta_d] -> Gain7/1
  Product5/1 -> Gain3/1
  Integrator3/1 -> Quantizer2/1, [alpha]  "alpha"
  Fcn5/1 -> Product5/1
  Product6/1 -> Gain4/1
  Sum2/1 -> Product4/1
  Math Function1/1 -> Product6/3
  Math Function/1 -> Product3/2
  Product/1 -> Integrator/1, [theta_dd]  "theta_dd"
  Gain4/1 -> Sum2/2
  Input_Voltage/1 -> Gain6/1
  Constant/1 -> Sum1/1
  [alpha] -> Fcn8/1, Fcn7/1, Fcn6/1, Fcn5/1
  Constant1/1 -> Product4/2
  Product2/1 -> Gain1/1
  [alpha] -> Fcn4/1, Fcn3/1, Fcn2/1, Fcn1/1
  [alpha_d] -> Product2/4
  [alpha_dd] -> Product1/2
  [alpha] -> Fcn/1
  Fcn2/1 -> Product2/1
  Sum3/1 -> Sum/4  "input torque"
  Gain2/1 -> Sum/3
  Gain/1 -> Sum/1
  Gain3/1 -> Sum2/1
  [theta_d] -> Math Function1/1
  Gain7/1 -> Sum3/2
  [theta_d] -> Product2/3
  Zero-Order Hold1/1 -> theta/1
  Quantizer2/1 -> Zero-Order Hold2/1
  Zero-Order Hold2/1 -> alpha/1
  Quantizer1/1 -> Zero-Order Hold1/1

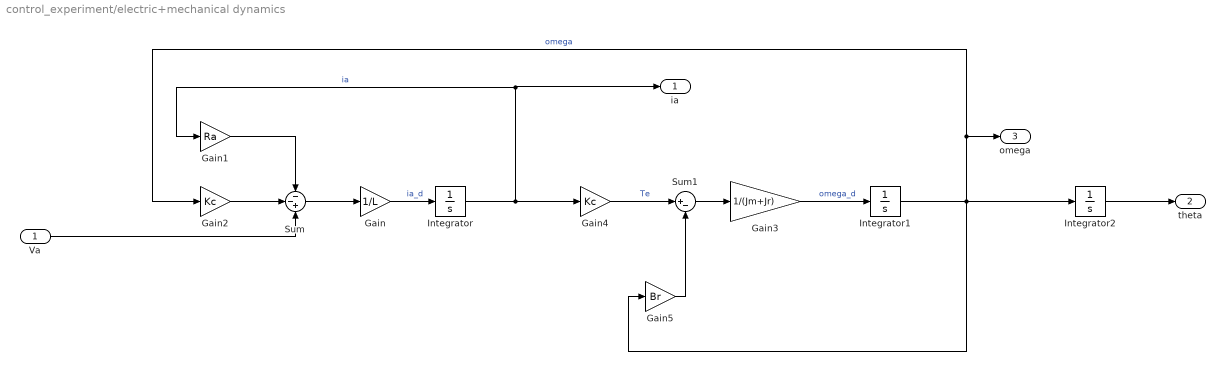
== system control_experiment/electric+mechanical dynamics ==
  Va : Inport
  Gain : Gain  Gain=1/L
  Gain1 : Gain  Gain=Ra
  Gain2 : Gain  Gain=Kc
  Gain3 : Gain  Gain=1/(Jm+Jr)
  Gain4 : Gain  Gain=Kc
  Gain5 : Gain  Gain=Br
  Integrator : Integrator
  Integrator1 : Integrator  InitialCondition=thetadot_0
  Integrator2 : Integrator  InitialCondition=theta_0
  Sum : Sum  Inputs=--+
  Sum1 : Sum  Inputs=|+-
  ia : Outport
  theta : Outport  Port=2
  omega : Outport  Port=3
  wires:
  Gain2/1 -> Sum/2
  Gain1/1 -> Sum/1
  Gain/1 -> Integrator/1  "ia_d"
  Gain4/1 -> Sum1/1  "Te"
  Gain5/1 -> Sum1/2
  Integrator1/1 -> omega/1, Gain2/1, Integrator2/1, Gain5/1  "omega"
  Integrator/1 -> Gain4/1, ia/1, Gain1/1  "ia"
  Sum/1 -> Gain/1
  Va/1 -> Sum/3
  Sum1/1 -> Gain3/1
  Gain3/1 -> Integrator1/1  "omega_d"
  Integrator2/1 -> theta/1
